simulink model "DA42_Validations"  (Simulink 7.5)
settings: Solver=ode3  StartTime=0.0  StopTime=fdata(end,1)  FixedStep=0.02  RelTol=1e-3
undefined symbols (not defined in the file or in its folder): BHP_A, BHP_B, CP_norm, elebias, fdata, initalt, initbank, initeast, inithead, initnorth, initp, initpitch, initq, initr, initu, initv, initw, mapbias, Pr_Alt, PropEff_norm
libraries: simulink_extras x4, aerolibatmos2 x2
(part 1 of 2)
settings Model: Creator=eagle  LastModifiedBy=eagle

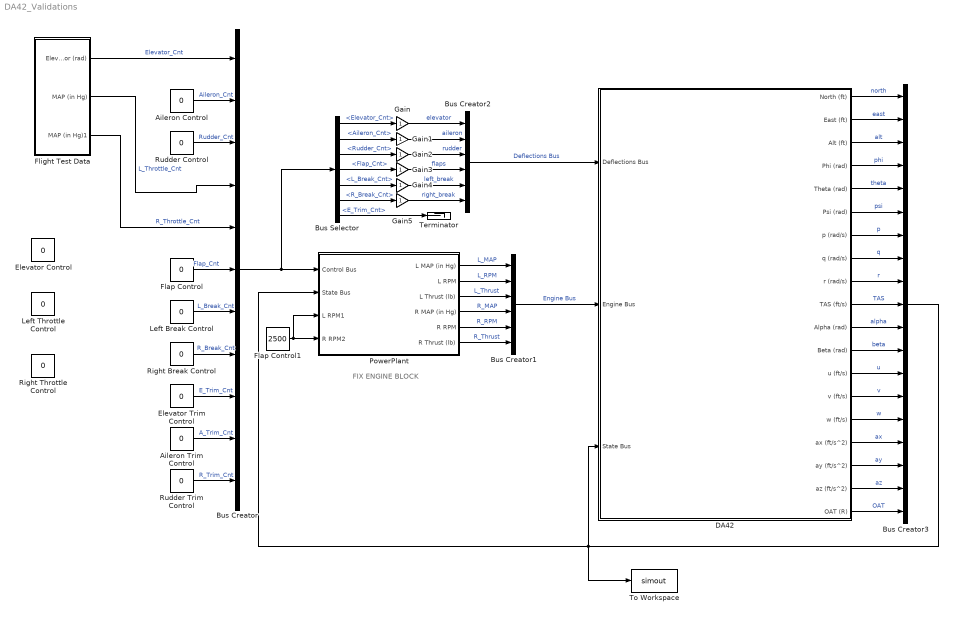
== system DA42_Validations ==
  note: FIX ENGINE BLOCK
  Aileron Control : Constant  Value=0  OutDataType=sfix(16)  OutScaling=2^0
  Aileron Trim Control : Constant  Value=0  OutDataType=sfix(16)  OutScaling=2^0
  Bus Creator : BusCreator  Inputs='Elevator_Cnt','Aileron_Cnt','Rudder_Cnt','L_Throttle_Cnt','R_Throttle_Cnt','Flap_Cnt','L_Break_Cnt','R_Break_Cnt','E_Trim_Cnt','A_Trim_Cnt','R_Trim_Cnt'
  Bus Creator1 : BusCreator  Inputs='L_MAP','L_RPM','L_Thrust','R_MAP','R_RPM','R_Thrust'
  Bus Creator2 : BusCreator  Inputs='elevator','aileron','rudder','flaps','left_break','right_break'
  Bus Creator3 : BusCreator  Inputs='north','east','alt','phi','theta','psi','p','q','r','TAS','alpha','beta','u','v','w','ax','ay','az','OAT'
  Bus Selector : BusSelector  OutputSignals=Elevator_Cnt,Aileron_Cnt,Rudder_Cnt,Flap_Cnt,L_Break_Cnt,R_Break_Cnt,E_Trim_Cnt
  DA42 : Subsystem
  Elevator Control : Constant  Value=0  OutDataType=sfix(16)  OutScaling=2^0
  Elevator Trim Control : Constant  Value=0  OutDataType=sfix(16)  OutScaling=2^0
  Flap Control : Constant  Value=0  OutDataType=sfix(16)  OutScaling=2^0
  Flap Control1 : Constant  Value=2500  OutDataType=sfix(16)  OutScaling=2^0
  Flight Test Data : Subsystem
  Gain{,1..5} (6 alike) : Gain  ParameterDataType=fixdt(1, 16)  ParameterScaling=2^0  OutDataType=fixdt(1, 16)  OutScaling=2^0
  Left Break Control : Constant  Value=0  OutDataType=sfix(16)  OutScaling=2^0
  Left Throttle Control : Constant  Value=0  OutDataType=sfix(16)  OutScaling=2^0
  PowerPlant : Subsystem  InitFcn=|
      | pitch_Angles = 15:5:40;
      | newData1 = load('-mat', 'CP_norm');
      | % Create new variables in the base workspace from those fields.
      | vars = fieldnames(newData1);
      | for i = 1:length(vars)
      |     assignin('base', vars{i}, newData1.(vars{i}));
      | end
      | clear i newData1 vars;
      | newData1 = load('-mat', 'PropEff_norm');
      | % Create new variables in the base workspace from those fields.
      | vars = fieldnames(newData1);
      | for i = 1:length(vars)
      |     assignin('base', vars{i}, newData1.(vars{i}));
      | end
      | clear i newData1 vars;
      | %% Lycoming IO-360 ENGINE PERFORMANCE
      | MAP = 12:2:28;
      | RPM = [2000; 2200; 2400; 2600; 2700];
      | %Table1:
      |     %Known: MAP and RPM.
      |     %Output: BHP-A
      |     BHP_A = [...
      |          58.0,  65.0,  68.0,  69.7,  71.5;...
      |          67.0,  75.5,  80.5,  85.0,  86.0;...
      |          79.0,  86.0,  92.5,  97.0,  99.0;...
      |          89.0,  97.0, 105.0, 110.5, 114.5;...
      |          98.0, 108.0, 116.0, 124.0, 126.0;...
      |         108.5, 118.5, 127.0, 135.5, 139.8;...
      |         118.0, 128.0, 139.0, 148.0, 152.5;...
      |         128.0, 139.0, 149.0, 160.0, 165.0;...
      |         137.5, 148.5, 161.0, 172.0, 177.5;...
      |         ];
      | %Table 2:
      |     %Known: MAP and RPM
      |     %Output: BHP-B
      |     %Comments: Equations for the lines based on linear extrapolation for
      |     %BHP-B. Has associated Excel File: "BHB_B.xlsx" to figure out the
      |     %equations for the lines
      |     for i = 1:9
      |         BHP_B(i,:) = [...
      |             ((6.818*MAP(i)) - 55.91),...
      |             ((7.167*MAP(i)) - 55.67),...
      |             ((7.857*MAP(i)) - 62.86),...
      |             ((8.333*MAP(i)) - 63.33),...
      |             ((8.5*MAP(i)) - 63),...
      |             ];
      |     end
      |     clear i;
      | %Table 3:
      |     %Known: MAP and RPM
      |     %Output: Pressure Altitude - A
      |     Pr_Alt = [...
      |         22.80, 22.70, 26.00, 25.00, 25.00;...
      |         19.20, 19.15, 19.10, 19.05, 19.00;...
      |         15.90, 15.80, 15.70, 15.60, 15.60;...
      |         12.95, 12.90, 12.80, 12.60, 12.55;...
      |         10.30, 10.25, 10.20, 10.10, 10.05;...
      |          7.85,  7.75,  7.65,  7.55,  7.50;...
      |          5.50,  5.47,  5.30,  5.25,  5.20;...
      |          3.40,  3.30,  3.25,  3.20,  3.15;...
      |          1.30,  1.25,  1.20,  1.10,  1.05;...
      |         ];
      |     Pr_Alt = Pr_Alt * 1000;
  Right Break Control : Constant  Value=0  OutDataType=sfix(16)  OutScaling=2^0
  Right Throttle Control : Constant  Value=0  OutDataType=sfix(16)  OutScaling=2^0
  Rudder Control : Constant  Value=0  OutDataType=sfix(16)  OutScaling=2^0
  Rudder Trim Control : Constant  Value=0  OutDataType=sfix(16)  OutScaling=2^0
  Terminator : Terminator
  To Workspace : ToWorkspace  VariableName=simout  SampleTime=-1  SaveFormat=Structure
  wires:
  Aileron Control/1 -> Bus Creator/2  "Aileron_Cnt"
  Rudder Control/1 -> Bus Creator/3  "Rudder_Cnt"
  Flap Control/1 -> Bus Creator/6  "Flap_Cnt"
  Left Break Control/1 -> Bus Creator/7  "L_Break_Cnt"
  Right Break Control/1 -> Bus Creator/8  "R_Break_Cnt"
  Elevator Trim Control/1 -> Bus Creator/9  "E_Trim_Cnt"
  Aileron Trim Control/1 -> Bus Creator/10  "A_Trim_Cnt"
  Rudder Trim Control/1 -> Bus Creator/11  "R_Trim_Cnt"
  PowerPlant/1(L MAP (in Hg)) -> Bus Creator1/1  "L_MAP"
  PowerPlant/2(L RPM) -> Bus Creator1/2  "L_RPM"
  PowerPlant/3(L Thrust (lb)) -> Bus Creator1/3  "L_Thrust"
  PowerPlant/4(R MAP (in Hg)) -> Bus Creator1/4  "R_MAP"
  PowerPlant/5(R RPM) -> Bus Creator1/5  "R_RPM"
  PowerPlant/6(R Thrust (lb)) -> Bus Creator1/6  "R_Thrust"
  Bus Selector/1 -> Gain/1  "<Elevator_Cnt>"
  Bus Selector/2 -> Gain1/1  "<Aileron_Cnt>"
  Bus Selector/3 -> Gain2/1  "<Rudder_Cnt>"
  Bus Selector/5 -> Gain4/1  "<L_Break_Cnt>"
  Bus Selector/7 -> Terminator/1  "<E_Trim_Cnt>"
  Bus Creator2/1 -> DA42/1(Deflections Bus)  "Deflections Bus"
  Bus Creator1/1 -> DA42/2(Engine Bus)  "Engine Bus"
  DA42/1(North (ft)) -> Bus Creator3/1  "north"
  DA42/2(East (ft)) -> Bus Creator3/2  "east"
  DA42/3(Alt (ft)) -> Bus Creator3/3  "alt"
  DA42/4(Phi (rad)) -> Bus Creator3/4  "phi"
  DA42/5(Theta (rad)) -> Bus Creator3/5  "theta"
  DA42/6(Psi (rad)) -> Bus Creator3/6  "psi"
  DA42/7(p (rad/s)) -> Bus Creator3/7  "p"
  DA42/8(q (rad/s)) -> Bus Creator3/8  "q"
  DA42/9(r (rad/s)) -> Bus Creator3/9  "r"
  DA42/10(TAS (ft/s)) -> Bus Creator3/10  "TAS"
  DA42/11(Alpha (rad)) -> Bus Creator3/11  "alpha"
  DA42/12(Beta (rad)) -> Bus Creator3/12  "beta"
  DA42/13(u (ft/s)) -> Bus Creator3/13  "u"
  DA42/14(v (ft/s)) -> Bus Creator3/14  "v"
  DA42/15(w (ft/s)) -> Bus Creator3/15  "w"
  DA42/16(ax (ft/s^2)) -> Bus Creator3/16  "ax"
  DA42/17(ay (ft/s^2)) -> Bus Creator3/17  "ay"
  DA42/18(az (ft/s^2)) -> Bus Creator3/18  "az"
  Bus Creator3/1 -> DA42/3(State Bus), PowerPlant/2(State Bus), To Workspace/1
  Bus Creator/1 -> PowerPlant/1(Control Bus), Bus Selector/1
  DA42/19(OAT (R)) -> Bus Creator3/19  "OAT"
  Flap Control1/1 -> PowerPlant/4(R RPM2), PowerPlant/3(L RPM1)
  Bus Selector/4 -> Gain3/1  "<Flap_Cnt>"
  Bus Selector/6 -> Gain5/1  "<R_Break_Cnt>"
  Gain/1 -> Bus Creator2/1  "elevator"
  Gain1/1 -> Bus Creator2/2  "aileron"
  Gain2/1 -> Bus Creator2/3  "rudder"
  Gain3/1 -> Bus Creator2/4  "flaps"
  Gain4/1 -> Bus Creator2/5  "left_break"
  Gain5/1 -> Bus Creator2/6  "right_break"
  Flight Test Data/1(Elevator (rad)) -> Bus Creator/1  "Elevator_Cnt"
  Flight Test Data/2(MAP (in Hg)) -> Bus Creator/4  "L_Throttle_Cnt"
  Flight Test Data/3(MAP (in Hg)1) -> Bus Creator/5  "R_Throttle_Cnt"

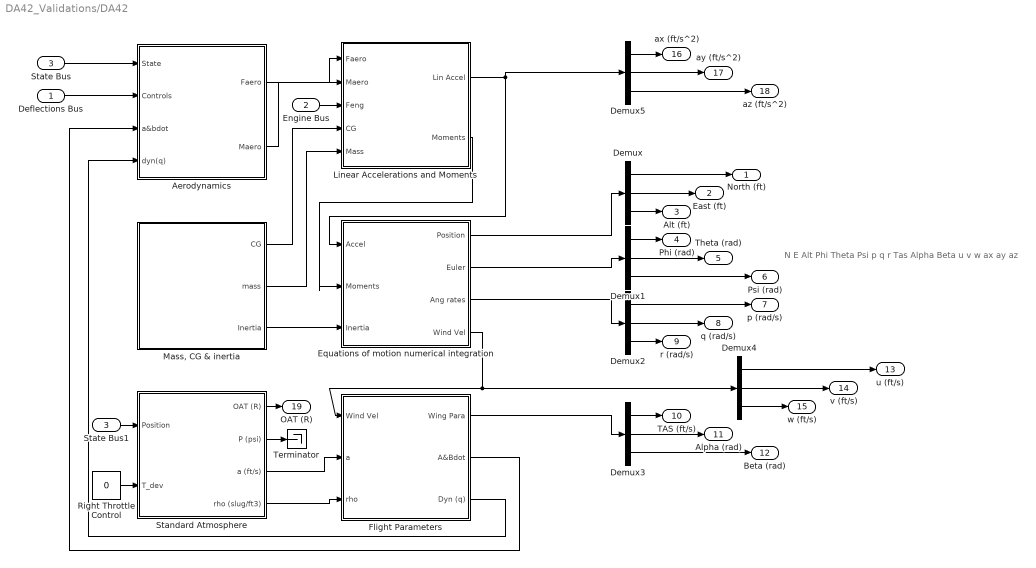
== system DA42_Validations/DA42 ==
  note: N
      | E
      | Alt
      | Phi
      | Theta
      | Psi
      | p
      | q
      | r
      | Tas
      | Alpha
      | Beta
      | u
      | v
      | w
      | ax
      | ay
      | az
  Deflections Bus : Inport
  Engine Bus : Inport  Port=2
  State Bus : Inport  Port=3
  Aerodynamics : Subsystem
  Demux{,1..5} (6 alike) : Demux  Outputs=3
  "Equations of motion numerical integration " : Subsystem
  Flight Parameters : Subsystem
  Linear Accelerations and Moments : Subsystem
  "Mass, CG & inertia" : Subsystem
  Right Throttle Control : Constant  Value=0  OutDataType=sfix(16)  OutScaling=2^0
  Standard Atmosphere : Subsystem
  State Bus1 : InportShadow  Port=3
  Terminator : Terminator
  North (ft) : Outport
  East (ft) : Outport  Port=2
  Alt (ft) : Outport  Port=3
  Phi (rad) : Outport  Port=4
  Theta (rad) : Outport  Port=5
  Psi (rad) : Outport  Port=6
  p (rad/s) : Outport  Port=7
  q (rad/s) : Outport  Port=8
  r (rad/s) : Outport  Port=9
  TAS (ft/s) : Outport  Port=10
  Alpha (rad) : Outport  Port=11
  Beta (rad) : Outport  Port=12
  u (ft/s) : Outport  Port=13
  v (ft/s) : Outport  Port=14
  w (ft/s) : Outport  Port=15
  ax (ft/s^2) : Outport  Port=16
  ay (ft/s^2) : Outport  Port=17
  az (ft/s^2) : Outport  Port=18
  OAT (R) : Outport  Port=19
  wires:
  "Equations of motion numerical integration "/1(Position) -> Demux/1
  Flight Parameters/2(A&Bdot) -> Aerodynamics/3(a&bdot)
  Flight Parameters/3(Dyn (q)) -> Aerodynamics/4(dyn(q))
  Flight Parameters/1(Wing Para) -> Demux3/1
  "Equations of motion numerical integration "/4(Wind Vel) -> Demux4/1, Flight Parameters/1(Wind Vel)
  "Equations of motion numerical integration "/3(Ang rates) -> Demux2/1
  Linear Accelerations and Moments/1(Lin Accel) -> "Equations of motion numerical integration "/1(Accel), Demux5/1
  Deflections Bus/1 -> Aerodynamics/2(Controls)
  Aerodynamics/2(Maero) -> Linear Accelerations and Moments/2(Maero)
  Aerodynamics/1(Faero) -> Linear Accelerations and Moments/1(Faero)
  Engine Bus/1 -> Linear Accelerations and Moments/3(Feng)
  Demux/1 -> North (ft)/1
  Demux/2 -> East (ft)/1
  Demux/3 -> Alt (ft)/1
  "Equations of motion numerical integration "/2(Euler) -> Demux1/1
  Demux1/1 -> Phi (rad)/1
  Demux1/2 -> Theta (rad)/1
  Demux1/3 -> Psi (rad)/1
  Demux2/1 -> p (rad/s)/1
  Demux2/2 -> q (rad/s)/1
  Demux2/3 -> r (rad/s)/1
  Demux3/1 -> TAS (ft/s)/1
  Demux3/2 -> Alpha (rad)/1
  Demux3/3 -> Beta (rad)/1
  Demux4/1 -> u (ft/s)/1
  Demux4/2 -> v (ft/s)/1
  Demux4/3 -> w (ft/s)/1
  Demux5/1 -> ax (ft/s^2)/1
  Demux5/2 -> ay (ft/s^2)/1
  Demux5/3 -> az (ft/s^2)/1
  Linear Accelerations and Moments/2(Moments) -> "Equations of motion numerical integration "/2(Moments)
  "Mass, CG & inertia"/1(CG) -> Linear Accelerations and Moments/4(CG)
  "Mass, CG & inertia"/2(mass) -> Linear Accelerations and Moments/5(Mass)
  "Mass, CG & inertia"/3(Inertia) -> "Equations of motion numerical integration "/3(Inertia)
  Standard Atmosphere/4(rho (slug/ft3)) -> Flight Parameters/3(rho)
  Standard Atmosphere/3(a (ft/s)) -> Flight Parameters/2(a)
  State Bus/1 -> Aerodynamics/1(State)
  State Bus1/1 -> Standard Atmosphere/1(Position)
  Standard Atmosphere/1(OAT (R)) -> OAT (R)/1
  Standard Atmosphere/2(P (psi)) -> Terminator/1
  Right Throttle Control/1 -> Standard Atmosphere/2(T_dev)

== system DA42_Validations/Flight Test Data ==
  Clock : Clock
      settings: Decimation=10
  Elevator : Lookup  InputValues=fdata(:,1)  Table=fdata(:,14)/57.3  OutDataType=fixdt(1, 16)  OutScaling=2^0
  Elevator Bias : Constant  Value=elebias  OutDataType=sfix(16)  OutScaling=2^0
  MAP : Lookup  InputValues=fdata(:,1)  Table=fdata(:,145)*0.000295301  OutDataType=fixdt(1, 16)  OutScaling=2^0
  MAP Bias : Constant  Value=mapbias  OutDataType=sfix(16)  OutScaling=2^0
  Sum : Sum  Inputs=|+-  OutDataType=fixdt(1, 16)  OutScaling=2^0
  Sum1 : Sum  Inputs=|+-  OutDataType=fixdt(1, 16)  OutScaling=2^0
  Elevator (rad) : Outport
  MAP (in Hg) : Outport  Port=2
  MAP (in Hg)1 : Outport  Port=3
  wires:
  Clock/1 -> Elevator/1, MAP/1
  Elevator/1 -> Sum/1
  Sum/1 -> Elevator (rad)/1
  Elevator Bias/1 -> Sum/2
  MAP/1 -> Sum1/1
  Sum1/1 -> MAP (in Hg)/1, MAP (in Hg)1/1
  MAP Bias/1 -> Sum1/2

== system DA42_Validations/PowerPlant ==
  Control Bus : Inport
  State Bus : Inport  Port=2
  L RPM1 : Inport  Port=3
  R RPM2 : Inport  Port=4
  Bus Selector : BusSelector  OutputSignals=L_Throttle_Cnt,R_Throttle_Cnt
  Bus Selector1 : BusSelector  OutputSignals=alt,OAT,TAS
  Bus Selector2 : BusSelector  OutputSignals=alt,OAT
  Lycoming IO-1 : Subsystem  InitFcn=|
      | pitch_Angles = 15:5:40;
      | newData1 = load('-mat', 'CP_norm');
      | % Create new variables in the base workspace from those fields.
      | vars = fieldnames(newData1);
      | for i = 1:length(vars)
      |     assignin('base', vars{i}, newData1.(vars{i}));
      | end
      | clear i newData1 vars;
      | newData1 = load('-mat', 'PropEff_norm');
      | % Create new variables in the base workspace from those fields.
      | vars = fieldnames(newData1);
      | for i = 1:length(vars)
      |     assignin('base', vars{i}, newData1.(vars{i}));
      | end
      | clear i newData1 vars;
      | %% Lycoming IO-360 ENGINE PERFORMANCE
      | MAP = 12:2:28;
      | RPM = [2000; 2200; 2400; 2600; 2700];
      | %Table1:
      |     %Known: MAP and RPM.
      |     %Output: BHP-A
      |     BHP_A = [...
      |          58.0,  65.0,  68.0,  69.7,  71.5;...
      |          67.0,  75.5,  80.5,  85.0,  86.0;...
      |          79.0,  86.0,  92.5,  97.0,  99.0;...
      |          89.0,  97.0, 105.0, 110.5, 114.5;...
      |          98.0, 108.0, 116.0, 124.0, 126.0;...
      |         108.5, 118.5, 127.0, 135.5, 139.8;...
      |         118.0, 128.0, 139.0, 148.0, 152.5;...
      |         128.0, 139.0, 149.0, 160.0, 165.0;...
      |         137.5, 148.5, 161.0, 172.0, 177.5;...
      |         ];
      | %Table 2:
      |     %Known: MAP and RPM
      |     %Output: BHP-B
      |     %Comments: Equations for the lines based on linear extrapolation for
      |     %BHP-B. Has associated Excel File: "BHB_B.xlsx" to figure out the
      |     %equations for the lines
      |     for i = 1:9
      |         BHP_B(i,:) = [...
      |             ((6.818*MAP(i)) - 55.91),...
      |             ((7.167*MAP(i)) - 55.67),...
      |             ((7.857*MAP(i)) - 62.86),...
      |             ((8.333*MAP(i)) - 63.33),...
      |             ((8.5*MAP(i)) - 63),...
      |             ];
      |     end
      |     clear i;
      | %Table 3:
      |     %Known: MAP and RPM
      |     %Output: Pressure Altitude - A
      |     Pr_Alt = [...
      |         22.80, 22.70, 26.00, 25.00, 25.00;...
      |         19.20, 19.15, 19.10, 19.05, 19.00;...
      |         15.90, 15.80, 15.70, 15.60, 15.60;...
      |         12.95, 12.90, 12.80, 12.60, 12.55;...
      |         10.30, 10.25, 10.20, 10.10, 10.05;...
      |          7.85,  7.75,  7.65,  7.55,  7.50;...
      |          5.50,  5.47,  5.30,  5.25,  5.20;...
      |          3.40,  3.30,  3.25,  3.20,  3.15;...
      |          1.30,  1.25,  1.20,  1.10,  1.05;...
      |         ];
      |     Pr_Alt = Pr_Alt * 1000;
  Lycoming IO-360 : Subsystem  InitFcn=|
      | pitch_Angles = 15:5:40;
      | newData1 = load('-mat', 'CP_norm');
      | % Create new variables in the base workspace from those fields.
      | vars = fieldnames(newData1);
      | for i = 1:length(vars)
      |     assignin('base', vars{i}, newData1.(vars{i}));
      | end
      | clear i newData1 vars;
      | newData1 = load('-mat', 'PropEff_norm');
      | % Create new variables in the base workspace from those fields.
      | vars = fieldnames(newData1);
      | for i = 1:length(vars)
      |     assignin('base', vars{i}, newData1.(vars{i}));
      | end
      | clear i newData1 vars;
      | %% Lycoming IO-360 ENGINE PERFORMANCE
      | MAP = 12:2:28;
      | RPM = [2000; 2200; 2400; 2600; 2700];
      | %Table1:
      |     %Known: MAP and RPM.
      |     %Output: BHP-A
      |     BHP_A = [...
      |          58.0,  65.0,  68.0,  69.7,  71.5;...
      |          67.0,  75.5,  80.5,  85.0,  86.0;...
      |          79.0,  86.0,  92.5,  97.0,  99.0;...
      |          89.0,  97.0, 105.0, 110.5, 114.5;...
      |          98.0, 108.0, 116.0, 124.0, 126.0;...
      |         108.5, 118.5, 127.0, 135.5, 139.8;...
      |         118.0, 128.0, 139.0, 148.0, 152.5;...
      |         128.0, 139.0, 149.0, 160.0, 165.0;...
      |         137.5, 148.5, 161.0, 172.0, 177.5;...
      |         ];
      | %Table 2:
      |     %Known: MAP and RPM
      |     %Output: BHP-B
      |     %Comments: Equations for the lines based on linear extrapolation for
      |     %BHP-B. Has associated Excel File: "BHB_B.xlsx" to figure out the
      |     %equations for the lines
      |     for i = 1:9
      |         BHP_B(i,:) = [...
      |             ((6.818*MAP(i)) - 55.91),...
      |             ((7.167*MAP(i)) - 55.67),...
      |             ((7.857*MAP(i)) - 62.86),...
      |             ((8.333*MAP(i)) - 63.33),...
      |             ((8.5*MAP(i)) - 63),...
      |             ];
      |     end
      |     clear i;
      | %Table 3:
      |     %Known: MAP and RPM
      |     %Output: Pressure Altitude - A
      |     Pr_Alt = [...
      |         22.80, 22.70, 26.00, 25.00, 25.00;...
      |         19.20, 19.15, 19.10, 19.05, 19.00;...
      |         15.90, 15.80, 15.70, 15.60, 15.60;...
      |         12.95, 12.90, 12.80, 12.60, 12.55;...
      |         10.30, 10.25, 10.20, 10.10, 10.05;...
      |          7.85,  7.75,  7.65,  7.55,  7.50;...
      |          5.50,  5.47,  5.30,  5.25,  5.20;...
      |          3.40,  3.30,  3.25,  3.20,  3.15;...
      |          1.30,  1.25,  1.20,  1.10,  1.05;...
      |         ];
      |     Pr_Alt = Pr_Alt * 1000;
  State Bus1 : InportShadow  Port=2
  L MAP (in Hg) : Outport  OutDataType=fixdt(1, 16)  OutScaling=2^0
  L RPM : Outport  Port=2  OutDataType=fixdt(1, 16)  OutScaling=2^0
  L Thrust (lb) : Outport  Port=3  OutDataType=fixdt(1, 16)  OutScaling=2^0
  R MAP (in Hg) : Outport  Port=4  OutDataType=fixdt(1, 16)  OutScaling=2^0
  R RPM : Outport  Port=5  OutDataType=fixdt(1, 16)  OutScaling=2^0
  R Thrust (lb) : Outport  Port=6  OutDataType=fixdt(1, 16)  OutScaling=2^0
  wires:
  Control Bus/1 -> Bus Selector/1
  Bus Selector/1 -> Lycoming IO-360/1(MAP), L MAP (in Hg)/1  "<L_Throttle_Cnt>"
  Bus Selector/2 -> Lycoming IO-1/1(MAP), R MAP (in Hg)/1  "<R_Throttle_Cnt>"
  L RPM1/1 -> Lycoming IO-360/2(RPM), L RPM/1
  Lycoming IO-1/1(Thrust (lb)) -> R Thrust (lb)/1
  Lycoming IO-360/1(Thrust (lb)) -> L Thrust (lb)/1
  R RPM2/1 -> Lycoming IO-1/2(RPM), R RPM/1
  State Bus/1 -> Bus Selector1/1
  Bus Selector1/1 -> Lycoming IO-360/3(Pressure Alt (ft))  "<alt>"
  Bus Selector1/2 -> Lycoming IO-360/4(OAT (R))  "<OAT>"
  Bus Selector1/3 -> Lycoming IO-360/5(TAS (ft/s))  "<TAS>"
  State Bus1/1 -> Bus Selector2/1
  Bus Selector2/1 -> Lycoming IO-1/3(Pressure Alt (ft))  "<alt>"
  Bus Selector2/2 -> Lycoming IO-1/4(OAT (R))  "<OAT>"

== system DA42_Validations/DA42/Aerodynamics ==
  State : Inport
  Controls : Inport  Port=2
  a&bdot : Inport  Port=3
  dyn(q) : Inport  Port=4
  Aero Forces and Moments : Subsystem
  CD : Subsystem
  CL : Subsystem
  CM : Subsystem
  CN : Subsystem
  CY : Subsystem
  Controls1 : InportShadow  Port=2
  Croll : Subsystem
  State1 : InportShadow  Port=1
  a&bdot1 : InportShadow  Port=3
  Faero : Outport
  Maero : Outport  Port=2
  wires:
  Aero Forces and Moments/2(Maero) -> Maero/1
  Aero Forces and Moments/1(Faero) -> Faero/1
  dyn(q)/1 -> Aero Forces and Moments/1(dyn(q))
  CM/1(CM) -> Aero Forces and Moments/7(CM)
  CY/1(CY) -> Aero Forces and Moments/3(CY)
  Croll/1(Croll) -> Aero Forces and Moments/6(Croll)
  CN/1(CN) -> Aero Forces and Moments/8(CN)
  CD/1(CD) -> Aero Forces and Moments/2(CD)
  Controls/1 -> CM/1(Controls), CL/1(Controls)
  State/1 -> CM/3(State), CL/3(State), CD/1(State)
  CL/1(CL) -> Aero Forces and Moments/4(CL)
  a&bdot/1 -> CM/2(a&bdot)
  a&bdot1/1 -> CL/2(a&bdot)
  Controls1/1 -> CY/2(Controls), Croll/1(Controls), CN/1(Controls)
  State1/1 -> CY/1(State), Croll/2(State), CN/2(State), Aero Forces and Moments/5(State)

== system DA42_Validations/DA42/Equations of motion numerical integration  ==
  Accel : Inport
  Moments : Inport  Port=2
  Inertia : Inport  Port=3
  Flat Earth Navigation : Subsystem
  Force Equations : Subsystem
  Gravity Model : Subsystem
  Inert-body : Subsystem
  Kinematic Equiations : Subsystem
  Moment Equations : Subsystem
  Terminator : Terminator
  Terminator1 : Terminator
  Position : Outport
  Euler : Outport  Port=2
  Ang rates : Outport  Port=3
  Wind Vel : Outport  Port=4
  wires:
  Inert-body/1(NEDtoBC) -> Force Equations/4(NEDtoABC)
  Flat Earth Navigation/1(Position) -> Position/1
  Moments/1 -> Moment Equations/2(Moments)
  Gravity Model/1(Gravity) -> Force Equations/2(Gravity)
  Inertia/1 -> Moment Equations/1(Inertia)
  Accel/1 -> Force Equations/1(Accel)
  Force Equations/1(Lin Vel) -> Flat Earth Navigation/2(Velocity), Wind Vel/1
  Kinematic Equiations/1(Euler angles) -> Euler/1, Inert-body/1(Euler), Flat Earth Navigation/1(Euler Angles)
  Moment Equations/1(Ang Rates) -> Ang rates/1, Force Equations/3(Rates), Kinematic Equiations/1(Rates)
  Moment Equations/2(Ang Accel) -> Terminator/1
  Kinematic Equiations/2(Euler Rates) -> Terminator1/1

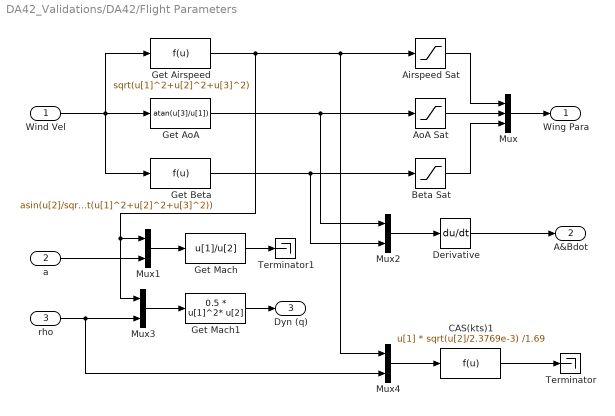
== system DA42_Validations/DA42/Flight Parameters ==
  Wind Vel : Inport
  a : Inport  Port=2
  rho : Inport  Port=3
  Airspeed Sat : Saturate  UpperLimit=1100  LowerLimit=0
  AoA Sat : Saturate  UpperLimit=0.3  LowerLimit=-0.2
  Beta Sat : Saturate  UpperLimit=0.4  LowerLimit=-0.4
  CAS(kts)1 : Fcn  Expr=u[1] * sqrt(u[2]/2.3769e-3) /1.69
  Derivative : Derivative
  Get Airspeed : Fcn  Expr=sqrt(u[1]^2+u[2]^2+u[3]^2)
  Get AoA : Fcn  Expr=atan(u[3]/u[1])
  Get Beta : Fcn  Expr=asin(u[2]/sqrt(u[1]^2+u[2]^2+u[3]^2))
  Get Mach : Fcn  Expr=u[1]/u[2]
  Get Mach1 : Fcn  Expr=0.5 * u[1]^2* u[2]
  Mux : Mux  Inputs=3
  Mux{1..4} (4 alike) : Mux  Inputs=2
  Terminator : Terminator
  Terminator1 : Terminator
  Wing Para : Outport
  A&Bdot : Outport  Port=2
  Dyn (q) : Outport  Port=3
  wires:
  Mux4/1 -> CAS(kts)1/1
  Get Mach1/1 -> Dyn (q)/1
  Mux3/1 -> Get Mach1/1
  rho/1 -> Mux4/2, Mux3/2
  Get Mach/1 -> Terminator1/1
  Derivative/1 -> A&Bdot/1
  Mux2/1 -> Derivative/1
  a/1 -> Mux1/2
  Mux1/1 -> Get Mach/1
  Mux/1 -> Wing Para/1
  Beta Sat/1 -> Mux/3
  Airspeed Sat/1 -> Mux/1
  AoA Sat/1 -> Mux/2
  Get Beta/1 -> Mux2/2, Beta Sat/1
  Get AoA/1 -> Mux2/1, AoA Sat/1
  Get Airspeed/1 -> Airspeed Sat/1, Mux4/1, Mux3/1, Mux1/1
  Wind Vel/1 -> Get Beta/1, Get Airspeed/1, Get AoA/1
  CAS(kts)1/1 -> Terminator/1

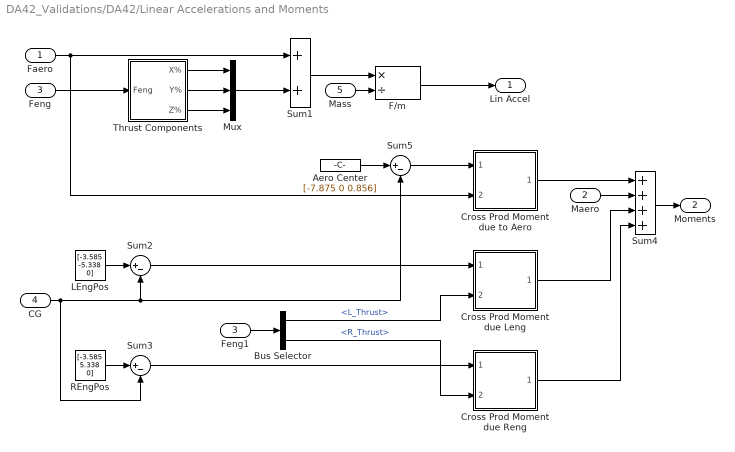
== system DA42_Validations/DA42/Linear Accelerations and Moments ==
  Faero : Inport
  Maero : Inport  Port=2
  Feng : Inport  Port=3
  CG : Inport  Port=4
  Mass : Inport  Port=5
  Aero Center : Constant  Value=[-7.875 0 0.856]
  Bus Selector : BusSelector  OutputSignals=L_Thrust,R_Thrust
  Cross Prod Moment due Leng : Subsystem
  Cross Prod Moment due Reng : Subsystem
  Cross Prod Moment due to Aero : Subsystem
  F/m : Product  Inputs=*/  SaturateOnIntegerOverflow=on  OutDataTypeStr=Inherit: Same as first input
  Feng1 : InportShadow  Port=3
  LEngPos : Constant  Value=[-3.585 -5.338 0]
  Mux : Mux  Inputs=3
  REngPos : Constant  Value=[-3.585 5.338 0]
  Sum1 : Sum  SaturateOnIntegerOverflow=on
  Sum2 : Sum  Inputs=|+-  SaturateOnIntegerOverflow=on
  Sum3 : Sum  Inputs=|+-  SaturateOnIntegerOverflow=on
  Sum4 : Sum  Inputs=++++  SaturateOnIntegerOverflow=on
  Sum5 : Sum  Inputs=|+-  SaturateOnIntegerOverflow=on
  Thrust Components : Subsystem
  Lin Accel : Outport
  Moments : Outport  Port=2
  wires:
  Cross Prod Moment due Reng/1(X Prod) -> Sum4/4
  Sum3/1 -> Cross Prod Moment due Reng/1(Vec 1)
  REngPos/1 -> Sum3/1
  LEngPos/1 -> Sum2/1
  Cross Prod Moment due Leng/1(X Prod) -> Sum4/3
  Sum2/1 -> Cross Prod Moment due Leng/1(Vec 1)
  Cross Prod Moment due to Aero/1(X Prod) -> Sum4/1
  Sum4/1 -> Moments/1
  Maero/1 -> Sum4/2
  Sum5/1 -> Cross Prod Moment due to Aero/1(Vec 1)
  Aero Center/1 -> Sum5/1
  CG/1 -> Sum3/2, Sum5/2, Sum2/2
  F/m/1 -> Lin Accel/1
  Mass/1 -> F/m/2
  Sum1/1 -> F/m/1
  Mux/1 -> Sum1/2
  Faero/1 -> Sum1/1, Cross Prod Moment due to Aero/2(Vec 2)
  Feng/1 -> Thrust Components/1(Feng)
  Thrust Components/1(X%) -> Mux/1
  Thrust Components/2(Y%) -> Mux/2
  Thrust Components/3(Z%) -> Mux/3
  Feng1/1 -> Bus Selector/1
  Bus Selector/1 -> Cross Prod Moment due Leng/2(Vec 2)  "<L_Thrust>"
  Bus Selector/2 -> Cross Prod Moment due Reng/2(Vec 2)  "<R_Thrust>"

== system DA42_Validations/DA42/Mass, CG & inertia ==
  Mux1 : Mux
  cg : Constant  Value=[-7.8750 0 0.856]
  jx : Constant  Value=6163.91
  jxz : Constant  Value=0
  jy : Constant  Value=1029.56
  jz : Constant  Value=5646.43
  mass2 : Constant  Value=3935/32.2
  CG : Outport
  mass : Outport  Port=2
  Inertia : Outport  Port=3
  wires:
  mass2/1 -> mass/1
  Mux1/1 -> Inertia/1
  jxz/1 -> Mux1/4
  jz/1 -> Mux1/3
  jx/1 -> Mux1/1
  jy/1 -> Mux1/2
  cg/1 -> CG/1

== system DA42_Validations/DA42/Standard Atmosphere ==
  note: From Aerospace Blockset
  Position : Inport  OutDataType=sfix(16)  OutScaling=2^0
  T_dev : Inport  Port=2  OutDataType=sfix(16)  OutScaling=2^0
  Atmosphere Model : Subsystem  mask(International Standard Atmosphere Model){custom=off, g=9.80665, gamma=1.4, R=287.0531, L=0.0065, h_trop=11000, h_strat=20000, rho0=1.225, P0=101325, T0=288.15}
      mask prompts: custom "Change atmospheric parameters"; g "Acceleration due to gravity (m/s^2):"; gamma "Ratio of specific heats:"; R "Characteristic gas constant (J/Kg/K):"; L "Lapse rate (K/m):"; h_trop "Height of troposphere (m):"; h_strat "Height of tropopause (m):"; rho0 "Air density at mean sea level (Kg/m^3):"; P0 "Ambient pressure at mean sea level (N/m^2):"; T0 "Ambient temperature at mean sea level (K):"
      mask help:
      | Compute International Standard Atmosphere (ISA) model for altitudes between 0 Km and 20 Km using a lapse rate method.
      |
      | Select change atmospheric parameters to create custom atmosphere.
      mask init:
      | ports = aeroicon('aeroblkisa','icon');
      | [x y miny txt] = aeroimage('atmosphere');
      mask Help: eval('asbhelp(''isa_atmosphere_model'')');
      mask CallbackString: aeroicon('aeroblkisa')|||||||||
      mask Display:
      | port_label('input',1,'h (m)','texmode','on');
      | port_label('output',1,'T (K)','texmode','on');
      | port_label('output',2,'a (m/s)','texmode','on');
      | port_label('output',3,'P (Pa)','texmode','on');
      | port_label('output',4,'\rho (kg/m^3)','texmode','on');
      | plot(x,y)
      | text(0.5,miny-.07,txt,'HorizontalAlignment','center');
  Bus Selector : BusSelector  OutputSignals=alt
  Kelvin 2 Rankine : Gain  Gain=1.8  ParameterDataType=sfix(16)  ParameterScaling=2^0  OutDataType=sfix(16)  OutScaling=2^0
  Pa 2 PSI : Gain  Gain=0.0001450377  ParameterDataType=sfix(16)  ParameterScaling=2^0  OutDataType=sfix(16)  OutScaling=2^0
  ft 2 m : Gain  Gain=0.3048  ParameterDataType=sfix(16)  ParameterScaling=2^0  OutDataType=sfix(16)  OutScaling=2^0
  kg/m3 2 slug/ft3 : Gain  Gain=0.00194032  ParameterDataType=sfix(16)  ParameterScaling=2^0  OutDataType=sfix(16)  OutScaling=2^0
  m/s 2 ft/s : Gain  Gain=3.280839895  ParameterDataType=sfix(16)  ParameterScaling=2^0  OutDataType=sfix(16)  OutScaling=2^0
  OAT (R) : Outport  OutDataType=sfix(16)  OutScaling=2^0
  P (psi) : Outport  Port=2  OutDataType=sfix(16)  OutScaling=2^0
  a (ft/s) : Outport  Port=3  OutDataType=sfix(16)  OutScaling=2^0
  rho (slug/ft3) : Outport  Port=4  OutDataType=sfix(16)  OutScaling=2^0
  wires:
  Position/1 -> Bus Selector/1
  Atmosphere Model/1(Temperature) -> Kelvin 2 Rankine/1
  Atmosphere Model/2(Speed of Sound) -> m/s 2 ft/s/1
  Atmosphere Model/4(Air Density) -> kg/m3 2 slug/ft3/1
  Atmosphere Model/3(Air Pressure) -> Pa 2 PSI/1
  ft 2 m/1 -> Atmosphere Model/1(Height)
  kg/m3 2 slug/ft3/1 -> rho (slug/ft3)/1
  Pa 2 PSI/1 -> P (psi)/1
  Kelvin 2 Rankine/1 -> OAT (R)/1
  T_dev/1 -> Atmosphere Model/2(Height1)
  m/s 2 ft/s/1 -> a (ft/s)/1
  Bus Selector/1 -> ft 2 m/1  "<alt>"

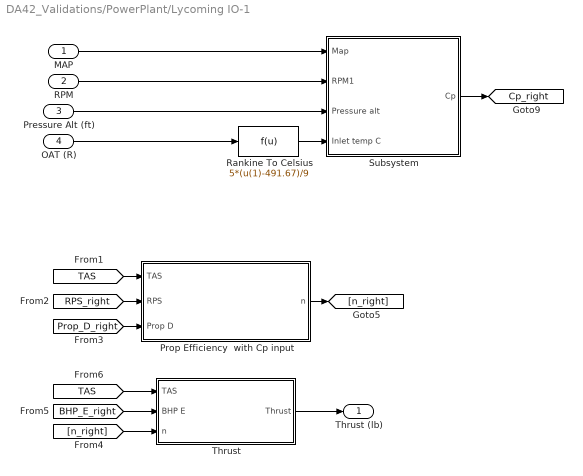
== system DA42_Validations/PowerPlant/Lycoming IO-1 ==
  MAP : Inport
  RPM : Inport  Port=2
  Pressure Alt (ft) : Inport  Port=3
  OAT (R) : Inport  Port=4
  Prop Efficiency  with Cp input : Subsystem
  Rankine To Celsius : Fcn  Expr=5*(u(1)-491.67)/9
  Subsystem : Subsystem
  Thrust : Subsystem
  Thrust (lb) : Outport
  tag scope: Cp_right=global
  wires:
  Thrust/1("Thrust ") -> Thrust (lb)/1
  Rankine To Celsius/1 -> Subsystem/4(Inlet temp C)
  OAT (R)/1 -> Rankine To Celsius/1
  Pressure Alt (ft)/1 -> Subsystem/3(Pressure alt)
  [TAS] -> Prop Efficiency  with Cp input/1(TAS)
  [RPS_right] -> Prop Efficiency  with Cp input/2(RPS)
  [Prop_D_right] -> Prop Efficiency  with Cp input/3(Prop D)
  [BHP_E_right] -> Thrust/2(BHP E)
  [n_right] -> Thrust/3(n)
  [TAS] -> Thrust/1(TAS)
  Prop Efficiency  with Cp input/1(n) -> [n_right]
  Subsystem/1(Cp) -> [Cp_right]
  MAP/1 -> Subsystem/1(Map)
  RPM/1 -> Subsystem/2(RPM1)

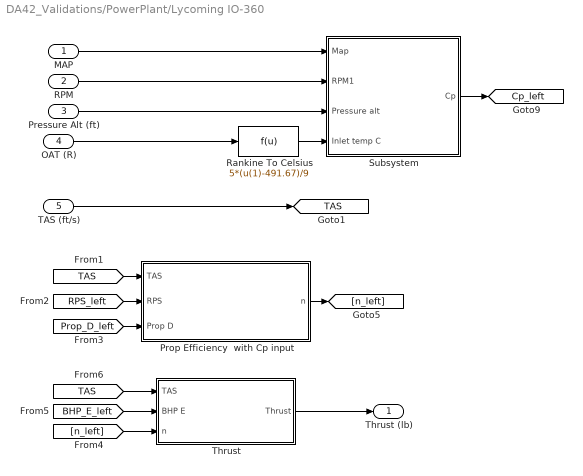
== system DA42_Validations/PowerPlant/Lycoming IO-360 ==
  MAP : Inport
  RPM : Inport  Port=2
  Pressure Alt (ft) : Inport  Port=3
  OAT (R) : Inport  Port=4
  TAS (ft/s) : Inport  Port=5
  Prop Efficiency  with Cp input : Subsystem
  Rankine To Celsius : Fcn  Expr=5*(u(1)-491.67)/9
  Subsystem : Subsystem
  Thrust : Subsystem
  Thrust (lb) : Outport
  tag scope: Cp_left=global, TAS=global
  wires:
  RPM/1 -> Subsystem/2(RPM1)
  MAP/1 -> Subsystem/1(Map)
  Subsystem/1(Cp) -> [Cp_left]
  Prop Efficiency  with Cp input/1(n) -> [n_left]
  [TAS] -> Thrust/1(TAS)
  [n_left] -> Thrust/3(n)
  [BHP_E_left] -> Thrust/2(BHP E)
  [Prop_D_left] -> Prop Efficiency  with Cp input/3(Prop D)
  [RPS_left] -> Prop Efficiency  with Cp input/2(RPS)
  [TAS] -> Prop Efficiency  with Cp input/1(TAS)
  Pressure Alt (ft)/1 -> Subsystem/3(Pressure alt)
  OAT (R)/1 -> Rankine To Celsius/1
  TAS (ft/s)/1 -> [TAS]
  Rankine To Celsius/1 -> Subsystem/4(Inlet temp C)
  Thrust/1("Thrust ") -> Thrust (lb)/1

== system DA42_Validations/DA42/Aerodynamics/Aero Forces and Moments ==
  dyn(q) : Inport
  CD : Inport  Port=2
  CY : Inport  Port=3
  CL : Inport  Port=4
  State : Inport  Port=5
  Croll : Inport  Port=6
  CM : Inport  Port=7
  CN : Inport  Port=8
  Aerodynamic Forces : Subsystem
  Aerodynamic Moments : Subsystem
  Faero : Outport
  Maero : Outport  Port=2
  wires:
  Aerodynamic Moments/1(Maero) -> Maero/1
  Aerodynamic Forces/1(FaeroBody) -> Faero/1
  CN/1 -> Aerodynamic Moments/4(CN)
  CM/1 -> Aerodynamic Moments/3(CM)
  Croll/1 -> Aerodynamic Moments/2(Croll)
  State/1 -> Aerodynamic Forces/4(State)
  CL/1 -> Aerodynamic Forces/3(CL)
  CY/1 -> Aerodynamic Forces/2(CY)
  CD/1 -> Aerodynamic Forces/1(CD)
  dyn(q)/1 -> Aerodynamic Forces/5(dyn(q)), Aerodynamic Moments/1(dyn(q))

== system DA42_Validations/DA42/Aerodynamics/CD ==
  State : Inport
  Bus Selector : BusSelector  OutputSignals=alpha
  Find Drag : Lookup_n-D  NumberOfTableDimensions=1  BreakpointsForDimension1="[-0.0986   -0.0828   -0.0654   -0.0511   -0.0312   -0.0179   -0.0084   -0.0003    0.0017    0.0064    0.0076    0.0099 0.0123    0.0157    0.0191    0.0207    0.0354    0.0487    0.0685    0.0828    0.1002    0.1161]"  Table="[0.0745    0.0652    0.0576    0.0528    0.0505    0.0502    0.0477    0.0475    0.0476    0.0475    0.0439    0.0435 0.0432    0.0432    0.0438    0.0485    0.0502    0.0505    0.0528    0.0576    0.0652    0.0745]"  RndMeth=Simplest  InputSameDT=on
  CD : Outport
  wires:
  Bus Selector/1 -> Find Drag/1  "<alpha>"
  State/1 -> Bus Selector/1
  Find Drag/1 -> CD/1

== system DA42_Validations/DA42/Aerodynamics/CL ==
  Controls : Inport
  a&bdot : Inport  Port=2
  State : Inport  Port=3
  "   7" : Terminator
  Bus Selector : BusSelector  OutputSignals=elevator
  Bus Selector1 : BusSelector  OutputSignals=alpha,q,TAS
  Demux2 : Demux  Outputs=2
  Fcn : Fcn  Expr=((u[1]+u[2])*4.17)/(2*u[3])
  Find CL : Lookup_n-D  NumberOfTableDimensions=1  BreakpointsForDimension1=[-0.26 0.13 0.533 0.991 2.03 2.474 2.96 3.6 4.059 4.45 5.335 5.38 5.5 5.84 6.19 6.569 7.12 7.54 7.92 8.42 8.71 9.29 9.74 10.34 11.176 12.238 13.249 13.605 13.921 14.753 15.482 15.911 16.682]/57.3  Table=[0.257 0.281 0.316 0.389 0.456 0.501 0.56 0.618 0.666 0.698 0.782 0.785 0.825 0.855 0.869 0.917 0.948 1.02 1.048 1.077 1.087 1.166 1.196 1.251 1.283 1.327 1.317 1.361 1.339 1.3066 1.28 1.244 1.195]  RndMeth=Simplest  InputSameDT=on
  Mux : Mux  Inputs=3
  Sum : Sum  Inputs=+++  SaturateOnIntegerOverflow=on
  cladot : Gain  Gain=0  SaturateOnIntegerOverflow=on  OutDataTypeStr=Inherit: Same as input  ParamDataTypeStr=Inherit: Same as input
  clde : Gain  Gain=0.7530  SaturateOnIntegerOverflow=on  OutDataTypeStr=Inherit: Same as input  ParamDataTypeStr=Inherit: Same as input
  clq : Gain  Gain=-41.807  SaturateOnIntegerOverflow=on  OutDataTypeStr=Inherit: Same as input  ParamDataTypeStr=Inherit: Same as input
  CL : Outport
  wires:
  clde/1 -> Sum/3
  clq/1 -> Mux/2
  cladot/1 -> Mux/1
  Demux2/1 -> cladot/1
  State/1 -> Bus Selector1/1
  a&bdot/1 -> Demux2/1
  Controls/1 -> Bus Selector/1
  Sum/1 -> CL/1
  Demux2/2 -> "   7"/1
  Mux/1 -> Fcn/1
  Find CL/1 -> Sum/1
  Fcn/1 -> Sum/2
  Bus Selector/1 -> clde/1  "<elevator>"
  Bus Selector1/1 -> Find CL/1  "<alpha>"
  Bus Selector1/2 -> clq/1  "<q>"
  Bus Selector1/3 -> Mux/3  "<TAS>"

== system DA42_Validations/DA42/Aerodynamics/CM ==
  Controls : Inport
  a&bdot : Inport  Port=2
  State : Inport  Port=3
  "   7" : Terminator
  Bus Selector : BusSelector  OutputSignals=elevator
  Bus Selector1 : BusSelector  OutputSignals=alpha,q,TAS
  Demux2 : Demux  Outputs=2
  Fcn : Fcn  Expr=((u[1]+u[2])*4.17)/(2*u[3])
  Mux : Mux  Inputs=3
  Sum : Sum  Inputs=+++  SaturateOnIntegerOverflow=on
  cma : Gain  Gain=-0.51  SaturateOnIntegerOverflow=on  OutDataTypeStr=Inherit: Same as input  ParamDataTypeStr=Inherit: Same as input
  cmadot : Gain  Gain=0  SaturateOnIntegerOverflow=on  OutDataTypeStr=Inherit: Same as input  ParamDataTypeStr=Inherit: Same as input
  cmde : Gain  Gain=-0.57  SaturateOnIntegerOverflow=on  OutDataTypeStr=Inherit: Same as input  ParamDataTypeStr=Inherit: Same as input
  cmq : Gain  Gain=-9.67  SaturateOnIntegerOverflow=on  OutDataTypeStr=Inherit: Same as input  ParamDataTypeStr=Inherit: Same as input
  CM : Outport
  wires:
  cmde/1 -> Sum/3
  Fcn/1 -> Sum/2
  Demux2/1 -> cmadot/1
  cma/1 -> Sum/1
  Mux/1 -> Fcn/1
  cmq/1 -> Mux/2
  cmadot/1 -> Mux/1
  State/1 -> Bus Selector1/1
  a&bdot/1 -> Demux2/1
  Controls/1 -> Bus Selector/1
  Sum/1 -> CM/1
  Demux2/2 -> "   7"/1
  Bus Selector/1 -> cmde/1  "<elevator>"
  Bus Selector1/1 -> cma/1  "<alpha>"
  Bus Selector1/2 -> cmq/1  "<q>"
  Bus Selector1/3 -> Mux/3  "<TAS>"

== system DA42_Validations/DA42/Aerodynamics/CN ==
  Controls : Inport
  State : Inport  Port=2
  Bus Selector : BusSelector  OutputSignals=aileron,rudder
  Bus Selector1 : BusSelector  OutputSignals=beta,alpha,p,r,TAS
  Divide : Product  Inputs=**
  Fcn : Fcn  Expr=((u[1]+u[2])*44)/(2*u[3])
  Find CNp : Lookup_n-D  NumberOfTableDimensions=1  BreakpointsForDimension1=[0 1 2 3 4 5 6 7 8]/57.3  Table=[-0.06 -0.078 -0.085 -0.095 -0.107 -0.119 -0.135 -0.14 -0.15]  RndMeth=Simplest  InputSameDT=on
  Mux : Mux  Inputs=3
  Sum : Sum  Inputs=++++  SaturateOnIntegerOverflow=on
  cnb : Gain  Gain=0.058  SaturateOnIntegerOverflow=on  OutDataTypeStr=Inherit: Same as input  ParamDataTypeStr=Inherit: Same as input
  cnda : Gain  Gain=-0.0033  SaturateOnIntegerOverflow=on  OutDataTypeStr=Inherit: Same as input  ParamDataTypeStr=Inherit: Same as input
  cndr : Gain  Gain=0.077  SaturateOnIntegerOverflow=on  OutDataTypeStr=Inherit: Same as input  ParamDataTypeStr=Inherit: Same as input
  cnr : Gain  Gain=-0.114  SaturateOnIntegerOverflow=on  OutDataTypeStr=Inherit: Same as input  ParamDataTypeStr=Inherit: Same as input
  CN : Outport
  wires:
  cndr/1 -> Sum/4
  cnda/1 -> Sum/3
  Fcn/1 -> Sum/2
  cnr/1 -> Mux/2
  cnb/1 -> Sum/1
  Controls/1 -> Bus Selector/1
  Sum/1 -> CN/1
  Mux/1 -> Fcn/1
  Find CNp/1 -> Divide/1
  Divide/1 -> Mux/1
  Bus Selector/1 -> cnda/1  "<aileron>"
  Bus Selector/2 -> cndr/1  "<rudder>"
  State/1 -> Bus Selector1/1
  Bus Selector1/1 -> cnb/1  "<beta>"
  Bus Selector1/2 -> Find CNp/1  "<alpha>"
  Bus Selector1/3 -> Divide/2  "<p>"
  Bus Selector1/4 -> cnr/1  "<r>"
  Bus Selector1/5 -> Mux/3  "<TAS>"

== system DA42_Validations/DA42/Aerodynamics/CY ==
  State : Inport
  Controls : Inport  Port=2
  Bus Selector : BusSelector  OutputSignals=rudder
  Bus Selector1 : BusSelector  OutputSignals=beta
  Sum : Sum  SaturateOnIntegerOverflow=on
  cyb : Gain  Gain=-0.28  SaturateOnIntegerOverflow=on  OutDataTypeStr=Inherit: Same as input  ParamDataTypeStr=Inherit: Same as input
  cydr : Gain  Gain=-0.3940  SaturateOnIntegerOverflow=on  OutDataTypeStr=Inherit: Same as input  ParamDataTypeStr=Inherit: Same as input
  CY : Outport
  wires:
  cydr/1 -> Sum/2
  cyb/1 -> Sum/1
  Controls/1 -> Bus Selector/1
  Sum/1 -> CY/1
  Bus Selector/1 -> cydr/1  "<rudder>"
  State/1 -> Bus Selector1/1
  Bus Selector1/1 -> cyb/1  "<beta>"

== system DA42_Validations/DA42/Aerodynamics/Croll ==
  Controls : Inport
  State : Inport  Port=2
  Bus Selector : BusSelector  OutputSignals=aileron,rudder
  Bus Selector1 : BusSelector  OutputSignals=beta,alpha,p,r,TAS
  Divide : Product  Inputs=**
  Fcn1 : Fcn  Expr=((u[1]+u[2])*44)/(2*u[3])
  Find CLr : Lookup_n-D  NumberOfTableDimensions=1  BreakpointsForDimension1=[0 1 2 3 4 5 6 7 8]/57.3  Table=[0.15 0.25 0.32 0.33 0.35 0.35 0.4 0.42 0.45]  RndMeth=Simplest  InputSameDT=on
  Mux : Mux  Inputs=3
  Sum : Sum  Inputs=++++  SaturateOnIntegerOverflow=on
  clb : Gain  Gain=-0.13  SaturateOnIntegerOverflow=on  OutDataTypeStr=Inherit: Same as input  ParamDataTypeStr=Inherit: Same as input
  clda : Gain  Gain=-0.19  SaturateOnIntegerOverflow=on  OutDataTypeStr=Inherit: Same as input  ParamDataTypeStr=Inherit: Same as input
  cldr : Gain  Gain=-0.0095  SaturateOnIntegerOverflow=on  OutDataTypeStr=Inherit: Same as input  ParamDataTypeStr=Inherit: Same as input
  clp : Gain  Gain=-0.76  SaturateOnIntegerOverflow=on  OutDataTypeStr=Inherit: Same as input  ParamDataTypeStr=Inherit: Same as input
  Croll : Outport
  wires:
  cldr/1 -> Sum/4
  clda/1 -> Sum/3
  Fcn1/1 -> Sum/2
  clb/1 -> Sum/1
  clp/1 -> Mux/1
  State/1 -> Bus Selector1/1
  Controls/1 -> Bus Selector/1
  Sum/1 -> Croll/1
  Mux/1 -> Fcn1/1
  Find CLr/1 -> Divide/1
  Divide/1 -> Mux/2
  Bus Selector/1 -> clda/1  "<aileron>"
  Bus Selector/2 -> cldr/1  "<rudder>"
  Bus Selector1/1 -> clb/1  "<beta>"
  Bus Selector1/2 -> Find CLr/1  "<alpha>"
  Bus Selector1/3 -> clp/1  "<p>"
  Bus Selector1/5 -> Mux/3  "<TAS>"
  Bus Selector1/4 -> Divide/2  "<r>"

== system DA42_Validations/DA42/Equations of motion numerical integration /Flat Earth Navigation ==
  note: 1  roll
      | 2  pitch
      | 3  yaw
      | 4 u
      | 5 v
      | 6 w
  Euler Angles : Inport
  Velocity : Inport  Port=2
  Alt : Integrator  InitialCondition=initalt
  Alttitude Dot : Fcn  Expr=u[4] * sin(u[2]) - u[5] * sin(u[1]) * cos(u[2]) - u[6] * cos(u[1]) * cos(u[2])
  Demux : Demux  Outputs=3
  Demux1 : Demux  Outputs=3
  East : Integrator  InitialCondition=initeast
  East Dot : Fcn  Expr=u[4] * cos(u[2])* sin(u[3]) + u[5] * (cos(u[1])*cos(u[3]) + sin(u[1])*sin(u[2])*sin(u[3])) + u[6] * (-sin(u[1])*cos(u[3])+cos(u[1])*sin(u[2])*sin(u[3]))
  Mux : Mux  Inputs=6
  Mux1 : Mux  Inputs=3
  North : Integrator  InitialCondition=initnorth
  North Dot : Fcn  Expr=u[4] * cos(u[2]) * cos(u[3]) + u[5]*(-cos(u[1])*sin(u[3])+sin(u[1])*sin(u[2])*sin(u[3]))+u[6]*(sin(u[1])*sin(u[3])+cos(u[1])*sin(u[2])*cos(u[3]))
  Position : Outport
  wires:
  Mux1/1 -> Position/1
  Alt/1 -> Mux1/3
  North/1 -> Mux1/1
  East/1 -> Mux1/2
  Alttitude Dot/1 -> Alt/1
  North Dot/1 -> North/1
  East Dot/1 -> East/1
  Mux/1 -> North Dot/1, Alttitude Dot/1, East Dot/1
  Demux1/3 -> Mux/6
  Demux1/2 -> Mux/5
  Demux1/1 -> Mux/4
  Demux/3 -> Mux/3
  Demux/2 -> Mux/2
  Demux/1 -> Mux/1
  Velocity/1 -> Demux1/1
  Euler Angles/1 -> Demux/1

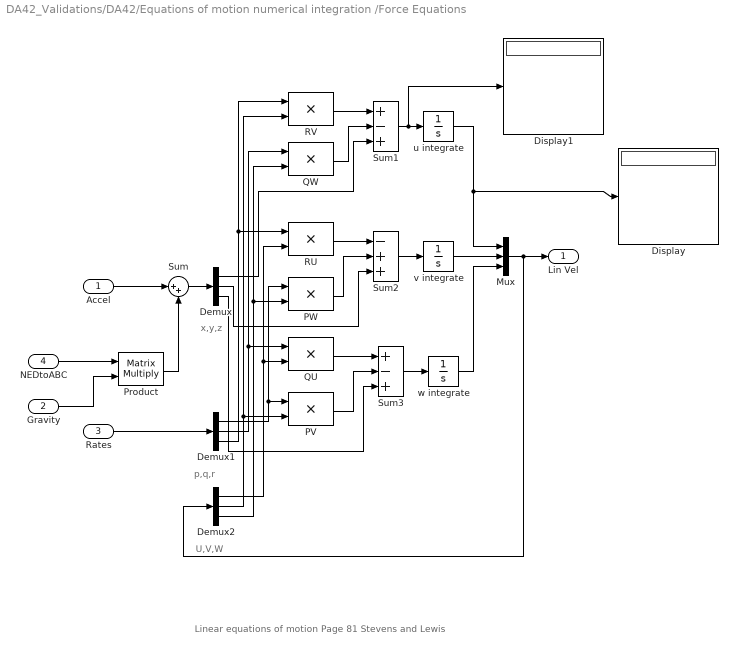
== system DA42_Validations/DA42/Equations of motion numerical integration /Force Equations ==
  note: Linear equations of motion
      | Page 81 Stevens and Lewis
  note: x,y,z
  note: p,q,r
  note: U,V,W
  Accel : Inport
  Gravity : Inport  Port=2
  Rates : Inport  Port=3
  NEDtoABC : Inport  Port=4
  Demux : Demux  Outputs=3
  Demux1 : Demux  Outputs=3
  Demux2 : Demux  Outputs=3
  Display : Display
  Display1 : Display
  Mux : Mux  Inputs=3
  PV : Product  SaturateOnIntegerOverflow=on  OutDataTypeStr=Inherit: Same as first input
  PW : Product  SaturateOnIntegerOverflow=on  OutDataTypeStr=Inherit: Same as first input
  Product : Product  Multiplication=Matrix(*)  SaturateOnIntegerOverflow=on  OutDataTypeStr=Inherit: Same as first input
  QU : Product  SaturateOnIntegerOverflow=on  OutDataTypeStr=Inherit: Same as first input
  QW : Product  SaturateOnIntegerOverflow=on  OutDataTypeStr=Inherit: Same as first input
  RU : Product  SaturateOnIntegerOverflow=on  OutDataTypeStr=Inherit: Same as first input
  RV : Product  SaturateOnIntegerOverflow=on  OutDataTypeStr=Inherit: Same as first input
  Sum : Sum  Inputs=|++  SaturateOnIntegerOverflow=on
  Sum1 : Sum  Inputs=+-+  SaturateOnIntegerOverflow=on
  Sum2 : Sum  Inputs=-++  SaturateOnIntegerOverflow=on
  Sum3 : Sum  Inputs=+-+  SaturateOnIntegerOverflow=on
  u integrate : Integrator  InitialCondition=initu
  v integrate : Integrator  InitialCondition=initv
  w integrate : Integrator  InitialCondition=initw
  Lin Vel : Outport
  wires:
  w integrate/1 -> Mux/3
  v integrate/1 -> Mux/2
  u integrate/1 -> Display/1, Mux/1
  Sum3/1 -> w integrate/1
  Sum2/1 -> v integrate/1
  Sum1/1 -> Display1/1, u integrate/1
  Product/1 -> Sum/2
  NEDtoABC/1 -> Product/1
  Gravity/1 -> Product/2
  Demux/3 -> Sum3/3
  PV/1 -> Sum3/2
  QU/1 -> Sum3/1
  Demux/2 -> Sum2/3
  PW/1 -> Sum2/2
  Demux1/1 -> PW/1, PV/1
  RU/1 -> Sum2/1
  Demux2/1 -> QU/2, RU/2
  Demux/1 -> Sum1/3
  QW/1 -> Sum1/2
  Demux2/3 -> PW/2, QW/2
  Demux1/2 -> QU/1, QW/1
  RV/1 -> Sum1/1
  Demux2/2 -> PV/2, RV/2
  Demux1/3 -> RU/1, RV/1
  Mux/1 -> Lin Vel/1, Demux2/1
  Rates/1 -> Demux1/1
  Accel/1 -> Sum/1
  Sum/1 -> Demux/1

== system DA42_Validations/DA42/Equations of motion numerical integration /Gravity Model ==
  Constant : Constant  Value=0
  Constant1 : Constant  Value=32.2
  Mux : Mux  Inputs=3
  Gravity : Outport
  wires:
  Mux/1 -> Gravity/1
  Constant1/1 -> Mux/3
  Constant/1 -> Mux/2, Mux/1

== system DA42_Validations/DA42/Equations of motion numerical integration /Inert-body ==
  Euler : Inport
  11 : Fcn  Expr=cos(u[2])*cos(u[3])
  12 : Fcn  Expr=-cos(u[1])*sin(u[3])+sin(u[1])*sin(u[2])*cos(u[3])
  13 : Fcn  Expr=sin(u[1])*sin(u[3])+cos(u[1])*sin(u[2])*cos(u[3])
  21 : Fcn  Expr=cos(u[2])*sin(u[3])
  22 : Fcn  Expr=cos(u[1])*cos(u[3]) + sin(u[1])*sin(u[2])*sin(u[3])
  23 : Fcn  Expr=-sin(u[1])*cos(u[3])+cos(u[1])*sin(u[2])*sin(u[3])
  31 : Fcn  Expr=-sin(u[2])
  32 : Fcn  Expr=sin(u[1]) * cos(u[2])
  33 : Fcn  Expr=cos(u[1])*cos(u[2])
  Matrix Concatenation : Concatenate  NumInputs=3  Mode=Multidimensional array
  Matrix Concatenation1 : Concatenate  NumInputs=3  Mode=Multidimensional array
  Matrix Concatenation2 : Concatenate  NumInputs=3  Mode=Multidimensional array
  Matrix Concatenation3 : Concatenate  NumInputs=3  Mode=Multidimensional array  ConcatenateDimension=2
  NEDtoBC : Outport
  wires:
  Matrix Concatenation3/1 -> NEDtoBC/1
  Matrix Concatenation2/1 -> Matrix Concatenation3/3
  Matrix Concatenation/1 -> Matrix Concatenation3/1
  Matrix Concatenation1/1 -> Matrix Concatenation3/2
  33/1 -> Matrix Concatenation2/3
  31/1 -> Matrix Concatenation2/1
  32/1 -> Matrix Concatenation2/2
  23/1 -> Matrix Concatenation1/3
  21/1 -> Matrix Concatenation1/1
  22/1 -> Matrix Concatenation1/2
  13/1 -> Matrix Concatenation/3
  11/1 -> Matrix Concatenation/1
  12/1 -> Matrix Concatenation/2
  Euler/1 -> 32/1, 33/1, 31/1, 23/1, 22/1, 21/1, 13/1, 12/1, 11/1

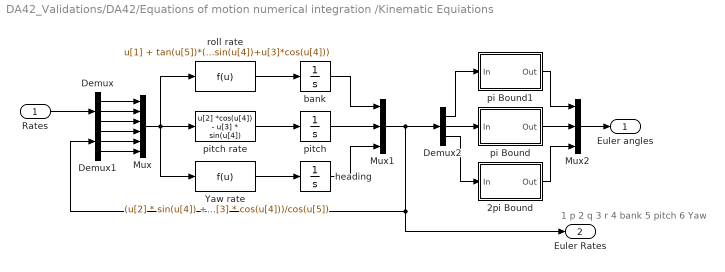
== system DA42_Validations/DA42/Equations of motion numerical integration /Kinematic Equiations ==
  note: 1  p
      | 2  q
      | 3  r
      | 4  bank
      | 5 pitch
      | 6 Yaw
  Rates : Inport
  2pi Bound : Subsystem
      mask Type: 2pi bound
      mask Description: Bounds the input angle to [0, 2pi]. When 0 bound is exceeded the output wraps back to 2pi; when the 2pi bound is exceeded the output wraps back to 0.
      mask Help:
      | Bounds the input angle to [0, 2pi]. When 0 bound is exceeded the output wraps back to 2pi; when the 2pi bound is exceeded the output wraps back to 0.
      | <P><B>Input:</B> any angle in radians, from -Inf to Inf;</P>
      | <P><B>Output:</B> an angle in radians between zero and 2pi.</P>
  Demux : Demux  Outputs=3
  Demux1 : Demux  Outputs=3
  Demux2 : Demux  Outputs=3
  Mux : Mux  Inputs=6
  Mux1 : Mux  Inputs=3
  Mux2 : Mux  Inputs=3
  Yaw rate : Fcn  Expr=(u[2] * sin(u[4]) + u[3] * cos(u[4]))/cos(u[5])
  bank : Integrator  InitialCondition=initbank
  heading : Integrator  InitialCondition=inithead
  pi Bound : Subsystem
      mask Type: pi bound
      mask Description: Bounds the input angle to [-pi, pi]. When -pi bound is exceeded the output wraps back to pi; when the pi bound is exceeded the output wraps back to -pi.
      mask Help:
      | Bounds the input angle to [-pi, pi]. When -pi bound is exceeded the output wraps back to pi; when the pi bound is exceeded the output wraps back to -pi.
      | <P><B>Input:</B> any angle in radians, from -Inf to Inf;</P>
      | <P><B>Output:</B> an angle in radians between -pi and pi.</P>
  pi Bound1 : Subsystem
      mask Type: pi bound
      mask Description: Bounds the input angle to [-pi, pi]. When -pi bound is exceeded the output wraps back to pi; when the pi bound is exceeded the output wraps back to -pi.
      mask Help:
      | Bounds the input angle to [-pi, pi]. When -pi bound is exceeded the output wraps back to pi; when the pi bound is exceeded the output wraps back to -pi.
      | <P><B>Input:</B> any angle in radians, from -Inf to Inf;</P>
      | <P><B>Output:</B> an angle in radians between -pi and pi.</P>
  pitch : Integrator  InitialCondition=initpitch
  pitch rate : Fcn  Expr=u[2] *cos(u[4]) - u[3] * sin(u[4])
  roll rate : Fcn  Expr=u[1] + tan(u[5])*(u[2]*sin(u[4])+u[3]*cos(u[4]))
  Euler angles : Outport
  Euler Rates : Outport  Port=2
  wires:
  Mux1/1 -> Euler Rates/1, Demux1/1, Demux2/1
  heading/1 -> Mux1/3
  pitch/1 -> Mux1/2
  bank/1 -> Mux1/1
  Yaw rate/1 -> heading/1
  roll rate/1 -> bank/1
  pitch rate/1 -> pitch/1
  2pi Bound/1(Out) -> Mux2/3
  pi Bound1/1(Out) -> Mux2/1
  pi Bound/1(Out) -> Mux2/2
  Mux2/1 -> Euler angles/1
  Demux2/1 -> pi Bound1/1(In)
  Demux2/2 -> pi Bound/1(In)
  Demux2/3 -> 2pi Bound/1(In)
  Mux/1 -> pitch rate/1, Yaw rate/1, roll rate/1
  Demux/1 -> Mux/1
  Demux1/3 -> Mux/6
  Demux1/2 -> Mux/5
  Demux1/1 -> Mux/4
  Demux/3 -> Mux/3
  Demux/2 -> Mux/2
  Rates/1 -> Demux/1

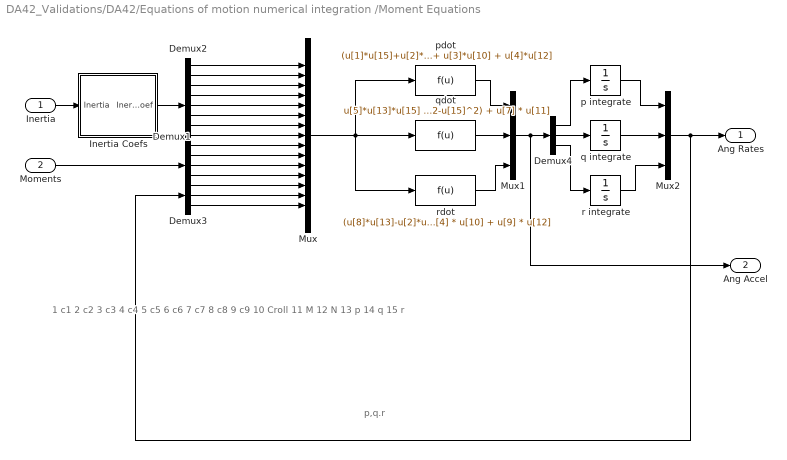
== system DA42_Validations/DA42/Equations of motion numerical integration /Moment Equations ==
  note: p,q.r
  note: 1   c1
      | 2   c2
      | 3   c3
      | 4  c4
      | 5  c5
      | 6  c6
      | 7  c7
      | 8  c8
      | 9  c9
      | 10 Croll
      | 11  M
      | 12  N
      | 13  p
      | 14  q
      | 15  r
  Inertia : Inport
  Moments : Inport  Port=2
  Demux1 : Demux  Outputs=3
  Demux2 : Demux  Outputs=9
  Demux3 : Demux  Outputs=3
  Demux4 : Demux  Outputs=3
  Inertia Coefs : Subsystem
  Mux : Mux  Inputs=15
  Mux1 : Mux  Inputs=3
  Mux2 : Mux  Inputs=3
  p integrate : Integrator  InitialCondition=initp
  pdot : Fcn  Expr=(u[1]*u[15]+u[2]*u[13])*u[14] + u[3]*u[10] + u[4]*u[12]
  q integrate : Integrator  InitialCondition=initq
  qdot : Fcn  Expr=u[5]*u[13]*u[15] - u[6]*(u[13]^2-u[15]^2) + u[7] * u[11]
  r integrate : Integrator  InitialCondition=initr
  rdot : Fcn  Expr=(u[8]*u[13]-u[2]*u[15]) * u[14] + u[4] * u[10] + u[9] * u[12]
  Ang Rates : Outport
  Ang Accel : Outport  Port=2
  wires:
  r integrate/1 -> Mux2/3
  q integrate/1 -> Mux2/2
  p integrate/1 -> Mux2/1
  Mux2/1 -> Demux3/1, Ang Rates/1
  Demux4/3 -> r integrate/1
  Demux4/2 -> q integrate/1
  Demux4/1 -> p integrate/1
  Mux1/1 -> Demux4/1, Ang Accel/1
  rdot/1 -> Mux1/3
  pdot/1 -> Mux1/1
  qdot/1 -> Mux1/2
  Mux/1 -> rdot/1, qdot/1, pdot/1
  Demux3/3 -> Mux/15
  Demux3/2 -> Mux/14
  Demux3/1 -> Mux/13
  Demux1/3 -> Mux/12
  Demux1/2 -> Mux/11
  Demux1/1 -> Mux/10
  Demux2/9 -> Mux/9
  Demux2/8 -> Mux/8
  Demux2/7 -> Mux/7
  Demux2/6 -> Mux/6
  Demux2/5 -> Mux/5
  Demux2/4 -> Mux/4
  Demux2/3 -> Mux/3
  Demux2/2 -> Mux/2
  Demux2/1 -> Mux/1
  Inertia Coefs/1(Iner Coef) -> Demux2/1
  Moments/1 -> Demux1/1
  Inertia/1 -> Inertia Coefs/1(Inertia)

== system DA42_Validations/DA42/Linear Accelerations and Moments/Cross Prod Moment due Leng ==
  Vec 1 : Inport
  Vec 2 : Inport  Port=2
  Check prob not zero : Constant  Value=0
  Demux : Demux  Outputs=3
  J axis : Fcn  Expr=u[4]*u[3] - u[6]*u[1]
  Mux : Mux  Inputs=6
  Mux1 : Mux  Inputs=3
  i axis : Fcn  Expr=u[6]*u[2] - u[5]*u[3]
  k axis : Fcn  Expr=u[5]*u[1] - u[4]*u[2]
  X Prod : Outport
  wires:
  Mux1/1 -> X Prod/1
  k axis/1 -> Mux1/3
  i axis/1 -> Mux1/1
  J axis/1 -> Mux1/2
  Mux/1 -> k axis/1, J axis/1, i axis/1
  Demux/2 -> Mux/2
  Demux/3 -> Mux/3
  Check prob not zero/1 -> Mux/6, Mux/5
  Demux/1 -> Mux/1
  Vec 1/1 -> Demux/1
  Vec 2/1 -> Mux/4

== system DA42_Validations/DA42/Linear Accelerations and Moments/Cross Prod Moment due Reng ==
  Vec 1 : Inport
  Vec 2 : Inport  Port=2
  Check prob not zero : Constant  Value=0
  Demux : Demux  Outputs=3
  J axis : Fcn  Expr=u[4]*u[3] - u[6]*u[1]
  Mux : Mux  Inputs=6
  Mux1 : Mux  Inputs=3
  i axis : Fcn  Expr=u[6]*u[2] - u[5]*u[3]
  k axis : Fcn  Expr=u[5]*u[1] - u[4]*u[2]
  X Prod : Outport
  wires:
  Mux1/1 -> X Prod/1
  k axis/1 -> Mux1/3
  i axis/1 -> Mux1/1
  J axis/1 -> Mux1/2
  Mux/1 -> k axis/1, J axis/1, i axis/1
  Demux/2 -> Mux/2
  Demux/3 -> Mux/3
  Check prob not zero/1 -> Mux/6, Mux/5
  Demux/1 -> Mux/1
  Vec 1/1 -> Demux/1
  Vec 2/1 -> Mux/4
